simulink model "drone_1"  (R2024a)
settings: Solver=VariableStepAuto  StartTime=0.0  StopTime=10  RelTol=1e-3
model workspace: external: MATLAB File E:\MIT notes\SEM 5\DL PROJECT\ED_Lab_Project\drone_DataFile1.m (data not in the file)
undefined symbols (not defined in the file or in its folder): smiData, X, Y, Z
libraries: sm_lib x30, nesl_utility x13, fl_lib x10, simulink x1
settings Model: Creator=CAPTMKPC  LastModifiedBy=CAPTMKPC
settings ExplorerConfigSet: InternalSimMechanicsExplorerSettings="<ExplorerConfiguration><canonicalview>aerospace</canonicalview><AnimationSetting><BasePlaybackSpeed>1.0</BasePlaybackSpeed><PlaybackSpeedFactor>1.0</PlaybackSpeedFactor></AnimationSetting><TilePanel><TileInfo><Tiles Columns=\"1\" Count=\"1\" Rows=\"1\"><Column Weight=\"1\"/><Row Weight=\"1\"/><Tile Height=\"1\" Width=\"1\" X=\"0\" Y=\"0\"/></Tiles></TileInfo><SceneInfo><SceneViewer><BGColor><R>0.60000002384185791</R><G>0.60000002384185791</G><B>0.60000002384185791</B></BGColor><Camera><DoPerspective>off</DoPerspective><Position><X>1.8589269016645551</X><Y>0.22741887211799594</Y><Z>-0.0186989009380337107</Z></Position><Center><X>0.00202931501269310033</X><Y>0.22741887211799594</Y><Z>-0.0186989009380337107</Z></Center><Up><X>0</X><Y>0</Y><Z>-1</Z></Up><ViewLimDist>1</ViewLimDist><YLim>0.859905762768950144</YLim><XLim>1.52803398132324242</XLim></Camera></SceneViewer></SceneInfo></TilePanel><MechEditorPanel><Cameras/><GfxPanelCameraMap/><VideoCreator><PlaybackSpeedRatio>1.0</PlaybackSpeedRatio><FrameRate>30</FrameRate><VideoFormat>Motion JPEG AVI</VideoFormat><FrameSize>auto</FrameSize></VideoCreator></MechEditorPanel></ExplorerConfiguration>"

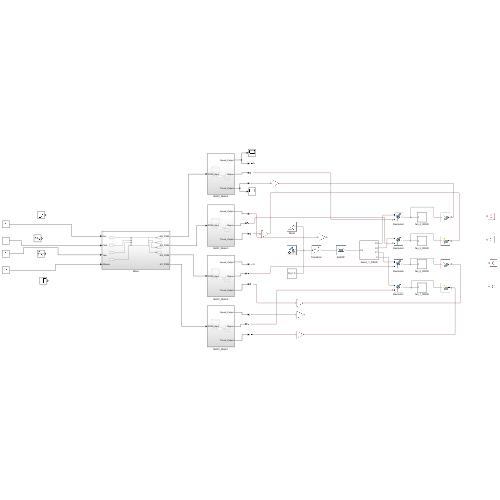
[thumbnail: Simulink's stored preview of the top-level diagram]
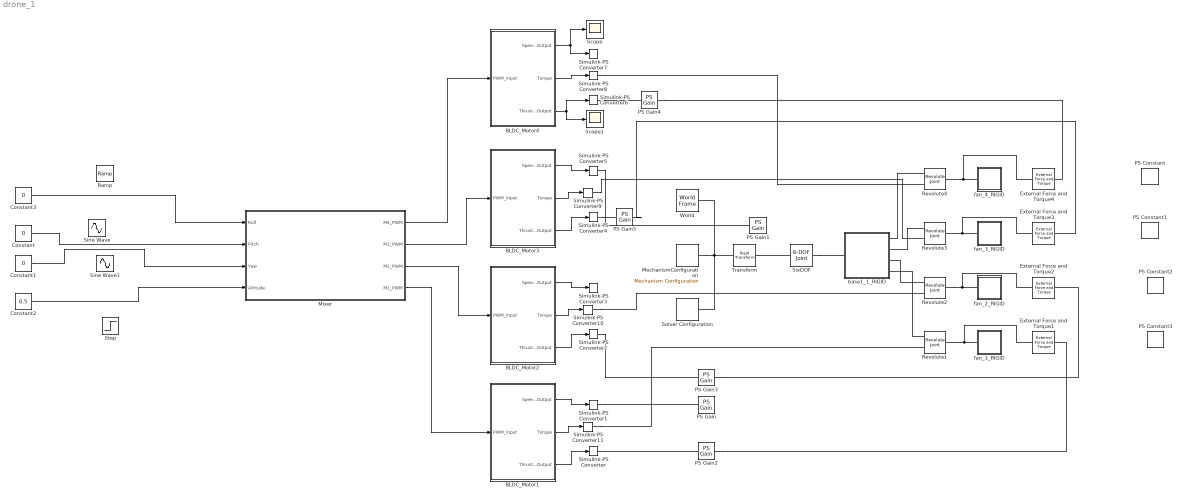
== system drone_1 ==
  BLDC_Motor1 : Subsystem
  BLDC_Motor2 : Subsystem
  BLDC_Motor3 : Subsystem
  BLDC_Motor4 : Subsystem
  Constant : Constant  Value=0
  Constant1 : Constant  Value=0
  Constant2 : Constant  Value=0.5
  Constant3 : Constant  Value=0
  External Force and Torque{1..4} (4 alike) : sm_lib/Forces and Torques/External Force and Torque  EnableForceX=off  EnableForceY=off  EnableForceZ=on  EnableForce=off  ForceResolutionFrame=World  EnableTorqueX=off  EnableTorqueY=off  EnableTorqueZ=off  EnableTorque=off  TorqueResolutionFrame=AttachedFrame
  MechanismConfiguration : sm_lib/Utilities/Mechanism Configuration  UniformGravity=Constant  GravityVector=[0 0 0]  GravityVectorUnits=m/s^2  LinearizationDelta=0.001  JointModeTransitionNonlinearIterations=2
  Mixer : Subsystem
  PS Constant{,1..3} (4 alike) : fl_lib/Physical Signals/Sources/PS Constant  constant=-308.4575 N
  PS Gain{,1..5} (6 alike) : fl_lib/Physical Signals/Functions/PS Gain  gain=-1
  Ramp : simulink/Sources/Ramp  slope=0.2  start=1  InitialOutput=0
  Revolute1 : sm_lib/Joints/Revolute Joint  JointMode=Normal  CompositeWrenchDir=FollowerOnBase  CompositeWrenchFrame=BaseFrame  SenseConstraintForce=off  SenseConstraintTorque=off  SenseTotalForce=off  SenseTotalTorque=off  PositionTargetSpecify=on  PositionTargetPriority=Low  PositionTargetValue=smiData.RevoluteJoint(1).Rz.Pos  PositionTargetValueUnits=deg  VelocityTargetSpecify=off  VelocityTargetPriority=High  VelocityTargetValue=0  VelocityTargetValueUnits=deg/s  EquilibriumPosition=0  EquilibriumPositionUnits=deg  SpringStiffness=0  SpringStiffnessUnits=N*m/deg  DampingCoefficient=0  DampingCoefficientUnits=N*m/(deg/s)  LowerLimitSpecify=off  LowerLimitBound=-90  LowerLimitBoundUnits=deg  LowerLimitStiffness=1e4  LowerLimitStiffnessUnits=N*m/deg  LowerLimitDamping=10  LowerLimitDampingUnits=N*m/(deg/s)  LowerLimitTransitionRegionWidth=0.1  LowerLimitTransitionRegionWidthUnits=deg  UpperLimitSpecify=off  UpperLimitBound=90  UpperLimitBoundUnits=deg  UpperLimitStiffness=1e4  UpperLimitStiffnessUnits=N*m/deg  UpperLimitDamping=10  UpperLimitDampingUnits=N*m/(deg/s)  UpperLimitTransitionRegionWidth=0.1  UpperLimitTransitionRegionWidthUnits=deg  TorqueActuationMode=InputTorque  MotionActuationMode=ComputedMotion  SensePosition=off  SenseVelocity=off  SenseAcceleration=off  SenseTorqueForce=off  SenseLowerLimitTorqueForce=off  SenseUpperLimitTorqueForce=off
  Revolute2 : sm_lib/Joints/Revolute Joint  JointMode=Normal  CompositeWrenchDir=FollowerOnBase  CompositeWrenchFrame=BaseFrame  SenseConstraintForce=off  SenseConstraintTorque=off  SenseTotalForce=off  SenseTotalTorque=off  PositionTargetSpecify=on  PositionTargetPriority=Low  PositionTargetValue=smiData.RevoluteJoint(2).Rz.Pos  PositionTargetValueUnits=deg  VelocityTargetSpecify=off  VelocityTargetPriority=High  VelocityTargetValue=0  VelocityTargetValueUnits=deg/s  EquilibriumPosition=0  EquilibriumPositionUnits=deg  SpringStiffness=0  SpringStiffnessUnits=N*m/deg  DampingCoefficient=0  DampingCoefficientUnits=N*m/(deg/s)  LowerLimitSpecify=off  LowerLimitBound=-90  LowerLimitBoundUnits=deg  LowerLimitStiffness=1e4  LowerLimitStiffnessUnits=N*m/deg  LowerLimitDamping=10  LowerLimitDampingUnits=N*m/(deg/s)  LowerLimitTransitionRegionWidth=0.1  LowerLimitTransitionRegionWidthUnits=deg  UpperLimitSpecify=off  UpperLimitBound=90  UpperLimitBoundUnits=deg  UpperLimitStiffness=1e4  UpperLimitStiffnessUnits=N*m/deg  UpperLimitDamping=10  UpperLimitDampingUnits=N*m/(deg/s)  UpperLimitTransitionRegionWidth=0.1  UpperLimitTransitionRegionWidthUnits=deg  TorqueActuationMode=InputTorque  MotionActuationMode=ComputedMotion  SensePosition=off  SenseVelocity=off  SenseAcceleration=off  SenseTorqueForce=off  SenseLowerLimitTorqueForce=off  SenseUpperLimitTorqueForce=off
  Revolute3 : sm_lib/Joints/Revolute Joint  JointMode=Normal  CompositeWrenchDir=FollowerOnBase  CompositeWrenchFrame=BaseFrame  SenseConstraintForce=off  SenseConstraintTorque=off  SenseTotalForce=off  SenseTotalTorque=off  PositionTargetSpecify=on  PositionTargetPriority=Low  PositionTargetValue=smiData.RevoluteJoint(3).Rz.Pos  PositionTargetValueUnits=deg  VelocityTargetSpecify=off  VelocityTargetPriority=High  VelocityTargetValue=0  VelocityTargetValueUnits=deg/s  EquilibriumPosition=0  EquilibriumPositionUnits=deg  SpringStiffness=0  SpringStiffnessUnits=N*m/deg  DampingCoefficient=0  DampingCoefficientUnits=N*m/(deg/s)  LowerLimitSpecify=off  LowerLimitBound=-90  LowerLimitBoundUnits=deg  LowerLimitStiffness=1e4  LowerLimitStiffnessUnits=N*m/deg  LowerLimitDamping=10  LowerLimitDampingUnits=N*m/(deg/s)  LowerLimitTransitionRegionWidth=0.1  LowerLimitTransitionRegionWidthUnits=deg  UpperLimitSpecify=off  UpperLimitBound=90  UpperLimitBoundUnits=deg  UpperLimitStiffness=1e4  UpperLimitStiffnessUnits=N*m/deg  UpperLimitDamping=10  UpperLimitDampingUnits=N*m/(deg/s)  UpperLimitTransitionRegionWidth=0.1  UpperLimitTransitionRegionWidthUnits=deg  TorqueActuationMode=InputTorque  MotionActuationMode=ComputedMotion  SensePosition=off  SenseVelocity=off  SenseAcceleration=off  SenseTorqueForce=off  SenseLowerLimitTorqueForce=off  SenseUpperLimitTorqueForce=off
  Revolute4 : sm_lib/Joints/Revolute Joint  JointMode=Normal  CompositeWrenchDir=FollowerOnBase  CompositeWrenchFrame=BaseFrame  SenseConstraintForce=off  SenseConstraintTorque=off  SenseTotalForce=off  SenseTotalTorque=off  PositionTargetSpecify=on  PositionTargetPriority=Low  PositionTargetValue=smiData.RevoluteJoint(4).Rz.Pos  PositionTargetValueUnits=deg  VelocityTargetSpecify=off  VelocityTargetPriority=High  VelocityTargetValue=0  VelocityTargetValueUnits=deg/s  EquilibriumPosition=0  EquilibriumPositionUnits=deg  SpringStiffness=0  SpringStiffnessUnits=N*m/deg  DampingCoefficient=0  DampingCoefficientUnits=N*m/(deg/s)  LowerLimitSpecify=off  LowerLimitBound=-90  LowerLimitBoundUnits=deg  LowerLimitStiffness=1e4  LowerLimitStiffnessUnits=N*m/deg  LowerLimitDamping=10  LowerLimitDampingUnits=N*m/(deg/s)  LowerLimitTransitionRegionWidth=0.1  LowerLimitTransitionRegionWidthUnits=deg  UpperLimitSpecify=off  UpperLimitBound=90  UpperLimitBoundUnits=deg  UpperLimitStiffness=1e4  UpperLimitStiffnessUnits=N*m/deg  UpperLimitDamping=10  UpperLimitDampingUnits=N*m/(deg/s)  UpperLimitTransitionRegionWidth=0.1  UpperLimitTransitionRegionWidthUnits=deg  TorqueActuationMode=InputTorque  MotionActuationMode=ComputedMotion  SensePosition=off  SenseVelocity=off  SenseAcceleration=off  SenseTorqueForce=off  SenseLowerLimitTorqueForce=off  SenseUpperLimitTorqueForce=off
  Scope : Scope
  Scope1 : Scope
  Simulink-PS Converter{,1..11} (12 alike) : nesl_utility/Simulink-PS Converter  PhysicalDomain=network_engine_domain  SubClassName=ps_input  LeftPortType=input  RightPortType=output  PseudoPeriodic=off  Frequencies=[]  NoiseDistribution=none  NoiseParameters=[]  Unit=1  AffineConversion=off  FilteringAndDerivatives=zero  SimscapeFilterOrder=1  InputFilterTimeConstant=0.001  UdotUserProvided=0
  Sine Wave : Sin  Amplitude=0.3  SampleTime=0
  Sine Wave1 : Sin  Amplitude=0.3  Frequency=0.5  Phase=90  SampleTime=0
  SixDOF : sm_lib/Joints/6-DOF Joint  JointMode=Normal  CompositeWrenchDir=FollowerOnBase  CompositeWrenchFrame=BaseFrame  SenseConstraintForce=off  SenseConstraintTorque=off  SenseTotalForce=off  SenseTotalTorque=off  PxPositionTargetSpecify=off  PxPositionTargetPriority=High  PxPositionTargetValue=0  PxPositionTargetValueUnits=m  PxVelocityTargetSpecify=off  PxVelocityTargetPriority=High  PxVelocityTargetValue=0  PxVelocityTargetValueUnits=m/s  PxEquilibriumPosition=0  PxEquilibriumPositionUnits=m  PxSpringStiffness=0  PxSpringStiffnessUnits=N/m  PxDampingCoefficient=0  PxDampingCoefficientUnits=N/(m/s)  PxLowerLimitSpecify=off  PxLowerLimitBound=-1  PxLowerLimitBoundUnits=m  PxLowerLimitStiffness=1e6  PxLowerLimitStiffnessUnits=N/m  PxLowerLimitDamping=1e3  PxLowerLimitDampingUnits=N/(m/s)  PxLowerLimitTransitionRegionWidth=1e-4  PxLowerLimitTransitionRegionWidthUnits=m  PxUpperLimitSpecify=off  PxUpperLimitBound=1  PxUpperLimitBoundUnits=m  PxUpperLimitStiffness=1e6  PxUpperLimitStiffnessUnits=N/m  PxUpperLimitDamping=1e3  PxUpperLimitDampingUnits=N/(m/s)  PxUpperLimitTransitionRegionWidth=1e-4  PxUpperLimitTransitionRegionWidthUnits=m  PxTorqueActuationMode=NoTorque  PxMotionActuationMode=ComputedMotion  PxSensePosition=off  PxSenseVelocity=off  PxSenseAcceleration=off  PxSenseTorqueForce=off  PxSenseLowerLimitTorqueForce=off  PxSenseUpperLimitTorqueForce=off  PyPositionTargetSpecify=off  PyPositionTargetPriority=High  PyPositionTargetValue=0  PyPositionTargetValueUnits=m  PyVelocityTargetSpecify=off  PyVelocityTargetPriority=High  PyVelocityTargetValue=0  PyVelocityTargetValueUnits=m/s  PyEquilibriumPosition=0  PyEquilibriumPositionUnits=m  PySpringStiffness=0  PySpringStiffnessUnits=N/m  PyDampingCoefficient=0  PyDampingCoefficientUnits=N/(m/s)  PyLowerLimitSpecify=off  PyLowerLimitBound=-1  PyLowerLimitBoundUnits=m  PyLowerLimitStiffness=1e6  PyLowerLimitStiffnessUnits=N/m  PyLowerLimitDamping=1e3  PyLowerLimitDampingUnits=N/(m/s)  PyLowerLimitTransitionRegionWidth=1e-4  PyLowerLimitTransitionRegionWidthUnits=m  PyUpperLimitSpecify=off  PyUpperLimitBound=1  PyUpperLimitBoundUnits=m  PyUpperLimitStiffness=1e6  PyUpperLimitStiffnessUnits=N/m  PyUpperLimitDamping=1e3  PyUpperLimitDampingUnits=N/(m/s)  PyUpperLimitTransitionRegionWidth=1e-4  PyUpperLimitTransitionRegionWidthUnits=m  PyTorqueActuationMode=NoTorque  PyMotionActuationMode=ComputedMotion  PySensePosition=off  PySenseVelocity=off  PySenseAcceleration=off  PySenseTorqueForce=off  PySenseLowerLimitTorqueForce=off  PySenseUpperLimitTorqueForce=off  PzPositionTargetSpecify=off  PzPositionTargetPriority=High  PzPositionTargetValue=0  PzPositionTargetValueUnits=m  PzVelocityTargetSpecify=off  PzVelocityTargetPriority=High  PzVelocityTargetValue=0  PzVelocityTargetValueUnits=m/s  PzEquilibriumPosition=0  PzEquilibriumPositionUnits=m  PzSpringStiffness=0  PzSpringStiffnessUnits=N/m  PzDampingCoefficient=0  PzDampingCoefficientUnits=N/(m/s)  PzLowerLimitSpecify=off  PzLowerLimitBound=-1  PzLowerLimitBoundUnits=m  PzLowerLimitStiffness=1e6  PzLowerLimitStiffnessUnits=N/m  PzLowerLimitDamping=1e3  PzLowerLimitDampingUnits=N/(m/s)  PzLowerLimitTransitionRegionWidth=1e-4  PzLowerLimitTransitionRegionWidthUnits=m  PzUpperLimitSpecify=off  PzUpperLimitBound=1  PzUpperLimitBoundUnits=m  PzUpperLimitStiffness=1e6  PzUpperLimitStiffnessUnits=N/m  PzUpperLimitDamping=1e3  PzUpperLimitDampingUnits=N/(m/s)  PzUpperLimitTransitionRegionWidth=1e-4  PzUpperLimitTransitionRegionWidthUnits=m  PzTorqueActuationMode=NoTorque  PzMotionActuationMode=ComputedMotion  PzSensePosition=off  PzSenseVelocity=off  PzSenseAcceleration=off  PzSenseTorqueForce=off  PzSenseLowerLimitTorqueForce=off  PzSenseUpperLimitTorqueForce=off  SphPositionTargetSpecify=off  SphPositionTargetPriority=High  SphPositionTargetRotationMethod=None  SphPositionTargetFollAlignAxisA=+X  SphPositionTargetBaseAlignAxisA=+Y  SphPositionTargetFollAlignAxisB=+Y  SphPositionTargetBaseAlignAxisB=+Z  SphPositionTargetRotationStandardAxis=+Z  SphPositionTargetRotationAngle=0  SphPositionTargetRotationAngleUnits=deg  SphPositionTargetRotationArbitraryAxis=[0 0 1]  SphPositionTargetRotationSequenceAxes=FollowerAxes  SphPositionTargetRotationSequence=XYX  SphPositionTargetRotationSequenceAngles=[0 0 0]  SphPositionTargetRotationSequenceAnglesUnits=deg  SphPositionTargetRotationMatrix=[1 0 0;0 1 0;0 0 1]  SphPositionTargetQuaternion=[1 0 0 0]  SphVelocityTargetSpecify=off  SphVelocityTargetPriority=High  SphVelocityTargetValue=[0 0 0]  SphVelocityTargetValueUnits=deg/s  SphVelocityTargetInFollowerFrame=on  SphEqPosRotationMethod=None  SphEqPosFollAlignAxisA=+X  SphEqPosBaseAlignAxisA=+Y  SphEqPosFollAlignAxisB=+Y  SphEqPosBaseAlignAxisB=+Z  SphEqPosRotationStandardAxis=+Z  SphEqPosRotationAngle=0  SphEqPosRotationAngleUnits=deg  SphEqPosRotationArbitraryAxis=[0 0 1]  SphEqPosRotationSequenceAxes=FollowerAxes  SphEqPosRotationSequence=XYX  SphEqPosRotationSequenceAngles=[0 0 0]  SphEqPosRotationSequenceAnglesUnits=deg  SphEqPosRotationMatrix=[1 0 0;0 1 0;0 0 1]  SphEqPosQuaternion=[1 0 0 0]  SphSpringStiffness=0  SphSpringStiffnessUnits=N*m/deg  SphDampingCoefficient=0  SphDampingCoefficientUnits=N*m/(deg/s)  SphLowerLimitSpecify=off  SphLowerLimitBound=15  SphLowerLimitBoundUnits=deg  SphLowerLimitStiffness=1e4  SphLowerLimitStiffnessUnits=N*m/deg  SphLowerLimitDamping=10  SphLowerLimitDampingUnits=N*m/(deg/s)  SphLowerLimitTransitionRegionWidth=0.1  SphLowerLimitTransitionRegionWidthUnits=deg  SphUpperLimitSpecify=off  SphUpperLimitBound=45  SphUpperLimitBoundUnits=deg  SphUpperLimitStiffness=1e4  SphUpperLimitStiffnessUnits=N*m/deg  SphUpperLimitDamping=10  SphUpperLimitDampingUnits=N*m/(deg/s)  SphUpperLimitTransitionRegionWidth=0.1  SphUpperLimitTransitionRegionWidthUnits=deg  SphTorqueActuationMode=NoTorque  SphActuateTorqueX=off  SphActuateTorqueY=off  SphActuateTorqueZ=off  SphActuateTorque=off  SphActuationFrame=BaseFrame  SphSensePosition=off  SphSenseVelocityX=off  SphSenseVelocityY=off  SphSenseVelocityZ=off  SphSenseVelocity=off  SphSenseAccelerationX=off  SphSenseAccelerationY=off  SphSenseAccelerationZ=off  SphSenseAcceleration=off  SphSenseLowerLimitTorqueMag=off  SphSenseUpperLimitTorqueMag=off  SphSensingFrame=FollowerFrame
  Solver Configuration : nesl_utility/Solver Configuration  PhysicalDomain=network_engine_domain  SubClassName=solver  LeftPortType=input  RightPortType=generic  Tones=[]  Harmonics=[]  SimulateNoise=off  Profile=off  UseLocalSampling=off  EnableSwitchedLinearOptims=on  FrequencyDomain=off  UseCCode=off  RelTol=0.001  AbsTol=0.001  MinStep=1e-09  ToWorkspace=off  RevertToSquareIcSolve=off  NumHomotopyIterations=100  PhasorMode=off  PhasorModeNumHarmonics=1  ConsistencySolver=NEWTON_XTOL_AFTER_FTOL  IndexReductionMethod=DerivativeReplacement  DoDC=off  ResidualTolerance=1e-09  ConsistencyTolSource=GLOBAL  ConsistencyAbsTol=0.001  ConsistencyRelTol=0.001  ConsistencyTolFactor=0.001  UseLocalSolver=off  LocalSolverChoice=NE_BACKWARD_EULER_ADVANCER  ResolveIndetEquations=on  FunctionEvalNumThread=1  LocalSolverSampleTime=0.001  DoFixedCost=off  MaxNonlinIter=3  MaxModeIter=2  ComputeImpulses=off  ImpulseIterations=2  LinearAlgebra=auto  LinearAlgebraNumThread=0  EquationFormulation=NE_TIME_EF  DelaysMemoryBudget=1024  AutomaticFiltering=on  FilteringTimeConstant=0.001  PartitionStorageMethod=AS_NEEDED  PartitionMemoryBudget=1024  PartitionMethod=ROBUST  MultibodyUseLocalSolver=off  MultibodyLocalSolverChoice=ODE1  MultibodyLocalSolverSampleTime=0.001
  Step : Step  Time=3  After=0.2  SampleTime=0
  Transform : sm_lib/Frames and Transforms/Rigid Transform  RotationMethod=StandardAxis  FollAlignAxisA=+X  BaseAlignAxisA=+Y  FollAlignAxisB=+Y  BaseAlignAxisB=+Z  RotationStandardAxis=+X  RotationAngle=-90  RotationAngleUnits=deg  RotationArbitraryAxis=smiData.RigidTransform(9).axis  RotationSequenceAxes=FollowerAxes  RotationSequence=XYX  RotationSequenceAngles=[0 0 0]  RotationSequenceAnglesUnits=deg  RotationMatrix=[1 0 0;0 1 0;0 0 1]  Quaternion=[1 0 0 0]  TranslationMethod=Cartesian  TranslationCartesianOffset=smiData.RigidTransform(9).translation  TranslationCartesianOffsetUnits=mm  TranslationStandardAxis=+Z  TranslationStandardOffset=0  TranslationStandardOffsetUnits=m  TranslationROffset=0  TranslationROffsetUnits=m  TranslationThetaOffset=0  TranslationThetaOffsetUnits=deg  TranslationZOffset=0  TranslationZOffsetUnits=m
  World : sm_lib/Frames and Transforms/World Frame
  base1_1_RIGID : Subsystem
  fan_1_RIGID : Subsystem
  fan_2_RIGID : Subsystem
  fan_3_RIGID : Subsystem
  fan_4_RIGID : Subsystem
  wires:
  BLDC_Motor4/1(Speed_Output) -> Simulink-PS Converter7/1, Scope/1
  BLDC_Motor4/3(Thrust_Output) -> Simulink-PS Converter6/1, Scope1/1
  Mixer/1(M4_PWM) -> BLDC_Motor4/1(PWM_Input)
  Constant3/1 -> Mixer/1(Roll)
  Constant/1 -> Mixer/2(Pitch)
  Constant1/1 -> Mixer/3(Yaw)
  Constant2/1 -> Mixer/4(Altitude)
  BLDC_Motor3/1(Speed_Output) -> Simulink-PS Converter5/1
  BLDC_Motor3/3(Thrust_Output) -> Simulink-PS Converter4/1
  BLDC_Motor2/1(Speed_Output) -> Simulink-PS Converter3/1
  BLDC_Motor2/3(Thrust_Output) -> Simulink-PS Converter2/1
  BLDC_Motor1/1(Speed_Output) -> Simulink-PS Converter1/1
  BLDC_Motor1/3(Thrust_Output) -> Simulink-PS Converter/1
  Mixer/2(M3_PWM) -> BLDC_Motor3/1(PWM_Input)
  Mixer/3(M2_PWM) -> BLDC_Motor2/1(PWM_Input)
  Mixer/4(M1_PWM) -> BLDC_Motor1/1(PWM_Input)
  BLDC_Motor4/2(Torque) -> Simulink-PS Converter8/1
  BLDC_Motor3/2(Torque) -> Simulink-PS Converter9/1
  BLDC_Motor2/2(Torque) -> Simulink-PS Converter10/1
  BLDC_Motor1/2(Torque) -> Simulink-PS Converter11/1
  connections:
  MechanismConfiguration/RConn1 -- Solver Configuration/RConn1 -- Transform/LConn1 -- World/RConn1
  Revolute1/LConn1 -- base1_1_RIGID/RConn4
  SixDOF/LConn1 -- Transform/RConn1
  Revolute1/RConn1 -- External Force and Torque1/RConn1 -- fan_1_RIGID/LConn1
  Revolute2/LConn1 -- base1_1_RIGID/RConn3
  Revolute2/RConn1 -- External Force and Torque2/RConn1 -- fan_2_RIGID/LConn1
  Revolute3/LConn1 -- base1_1_RIGID/RConn2
  Revolute3/RConn1 -- External Force and Torque3/RConn1 -- fan_3_RIGID/LConn1
  Revolute4/LConn1 -- base1_1_RIGID/RConn1
  Revolute4/RConn1 -- External Force and Torque4/RConn1 -- fan_4_RIGID/LConn1
  SixDOF/RConn1 -- base1_1_RIGID/LConn1
  Simulink-PS Converter6/RConn1 -- PS Gain4/LConn1
  Simulink-PS Converter4/RConn1 -- PS Gain5/LConn1
  Simulink-PS Converter2/RConn1 -- PS Gain3/LConn1
  Simulink-PS Converter/RConn1 -- PS Gain2/LConn1
  Simulink-PS Converter5/RConn1 -- PS Gain1/LConn1
  Simulink-PS Converter1/RConn1 -- PS Gain/LConn1
  PS Gain2/RConn1 -- External Force and Torque1/LConn1
  PS Gain3/RConn1 -- External Force and Torque2/LConn1
  PS Gain4/RConn1 -- External Force and Torque4/LConn1
  PS Gain5/RConn1 -- External Force and Torque3/LConn1
  Simulink-PS Converter8/RConn1 -- Revolute4/LConn2
  Simulink-PS Converter9/RConn1 -- Revolute3/LConn2
  Simulink-PS Converter10/RConn1 -- Revolute2/LConn2
  Simulink-PS Converter11/RConn1 -- Revolute1/LConn2

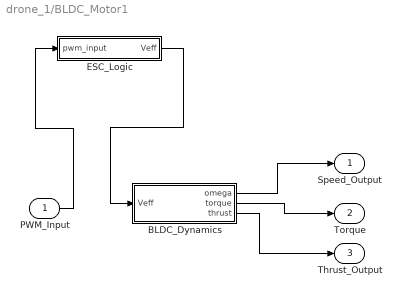
== system drone_1/BLDC_Motor1 ==
  PWM_Input : Inport
  BLDC_Dynamics : MATLAB Function  TreatAsAtomicUnit=on
  ESC_Logic : MATLAB Function  TreatAsAtomicUnit=on
  Speed_Output : Outport
  Torque : Outport  Port=2
  Thrust_Output : Outport  Port=3
  wires:
  BLDC_Dynamics/2(torque) -> Torque/1
  BLDC_Dynamics/1(omega) -> Speed_Output/1
  BLDC_Dynamics/3(thrust) -> Thrust_Output/1
  ESC_Logic/1(Veff) -> BLDC_Dynamics/1(Veff)
  PWM_Input/1 -> ESC_Logic/1(pwm_input)

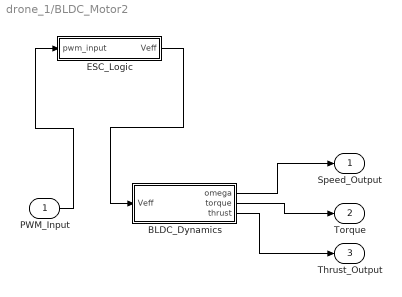
== system drone_1/BLDC_Motor2 ==
  PWM_Input : Inport
  BLDC_Dynamics : MATLAB Function  TreatAsAtomicUnit=on
  ESC_Logic : MATLAB Function  TreatAsAtomicUnit=on
  Speed_Output : Outport
  Torque : Outport  Port=2
  Thrust_Output : Outport  Port=3
  wires:
  BLDC_Dynamics/2(torque) -> Torque/1
  BLDC_Dynamics/1(omega) -> Speed_Output/1
  BLDC_Dynamics/3(thrust) -> Thrust_Output/1
  ESC_Logic/1(Veff) -> BLDC_Dynamics/1(Veff)
  PWM_Input/1 -> ESC_Logic/1(pwm_input)

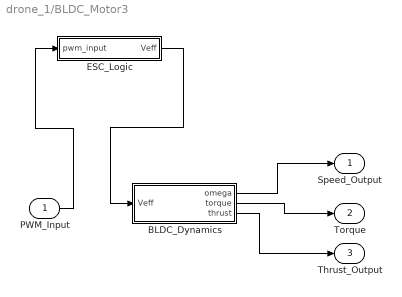
== system drone_1/BLDC_Motor3 ==
  PWM_Input : Inport
  BLDC_Dynamics : MATLAB Function  TreatAsAtomicUnit=on
  ESC_Logic : MATLAB Function  TreatAsAtomicUnit=on
  Speed_Output : Outport
  Torque : Outport  Port=2
  Thrust_Output : Outport  Port=3
  wires:
  BLDC_Dynamics/2(torque) -> Torque/1
  BLDC_Dynamics/1(omega) -> Speed_Output/1
  BLDC_Dynamics/3(thrust) -> Thrust_Output/1
  ESC_Logic/1(Veff) -> BLDC_Dynamics/1(Veff)
  PWM_Input/1 -> ESC_Logic/1(pwm_input)

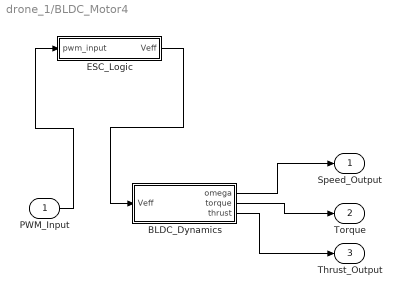
== system drone_1/BLDC_Motor4 ==
  PWM_Input : Inport
  BLDC_Dynamics : MATLAB Function  TreatAsAtomicUnit=on
  ESC_Logic : MATLAB Function  TreatAsAtomicUnit=on
  Speed_Output : Outport
  Torque : Outport  Port=2
  Thrust_Output : Outport  Port=3
  wires:
  ESC_Logic/1(Veff) -> BLDC_Dynamics/1(Veff)
  PWM_Input/1 -> ESC_Logic/1(pwm_input)
  BLDC_Dynamics/1(omega) -> Speed_Output/1
  BLDC_Dynamics/2(torque) -> Torque/1
  BLDC_Dynamics/3(thrust) -> Thrust_Output/1

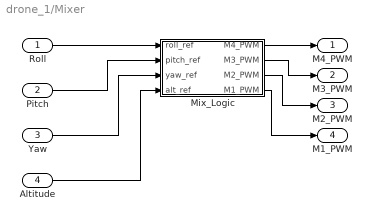
== system drone_1/Mixer ==
  Roll : Inport
  Pitch : Inport  Port=2
  Yaw : Inport  Port=3
  Altitude : Inport  Port=4
  Mix_Logic : MATLAB Function  TreatAsAtomicUnit=on
  M4_PWM : Outport
  M3_PWM : Outport  Port=2
  M2_PWM : Outport  Port=3
  M1_PWM : Outport  Port=4
  wires:
  Roll/1 -> Mix_Logic/1(roll_ref)
  Pitch/1 -> Mix_Logic/2(pitch_ref)
  Yaw/1 -> Mix_Logic/3(yaw_ref)
  Mix_Logic/1(M4_PWM) -> M4_PWM/1
  Mix_Logic/2(M3_PWM) -> M3_PWM/1
  Mix_Logic/3(M2_PWM) -> M2_PWM/1
  Mix_Logic/4(M1_PWM) -> M1_PWM/1
  Altitude/1 -> Mix_Logic/4(alt_ref)

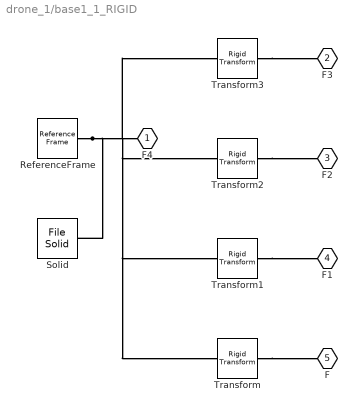
== system drone_1/base1_1_RIGID ==
  ReferenceFrame : sm_lib/Frames and Transforms/Reference Frame
  Solid : sm_lib/Body Elements/File Solid  ExtGeomFileName=base1_Default_sldprt.STEP  UnitType=FromFile  ExtGeomFileUnits=m  StepReaderType=HEX  ExportConvexHullGeometry=off  InertiaType=Custom  BasedOnType=DensityFromFile  Density=1000  DensityUnits=kg/m^3  Mass=smiData.Solid(1).mass  MassUnits=kg  CenterOfMass=smiData.Solid(1).CoM  CenterOfMassUnits=mm  MomentsOfInertia=smiData.Solid(1).MoI  MomentsOfInertiaUnits=kg*mm^2  ProductsOfInertia=smiData.Solid(1).PoI  ProductsOfInertiaUnits=kg*mm^2  GraphicType=FromGeometry  MarkerShape=Sphere  MarkerSize=10  GraphicVisPropType=SimpleVisualProperties  GraphicDiffuseColor=smiData.Solid(1).color  GraphicOpacity=smiData.Solid(1).opacity  GraphicSpecularColor=[0.5 0.5 0.5 1.0]  GraphicAmbientColor=[0.15 0.15 0.15 1.0]  GraphicEmissiveColor=[0.0 0.0 0.0 1.0]  GraphicShininess=75  DoExposeReferenceFrame=on  SerializedFrames=<Frames/>
  Transform : sm_lib/Frames and Transforms/Rigid Transform  RotationMethod=ArbitraryAxis  FollAlignAxisA=+X  BaseAlignAxisA=+Y  FollAlignAxisB=+Y  BaseAlignAxisB=+Z  RotationStandardAxis=+Z  RotationAngle=smiData.RigidTransform(1).angle  RotationAngleUnits=rad  RotationArbitraryAxis=smiData.RigidTransform(1).axis  RotationSequenceAxes=FollowerAxes  RotationSequence=XYX  RotationSequenceAngles=[0 0 0]  RotationSequenceAnglesUnits=deg  RotationMatrix=[1 0 0;0 1 0;0 0 1]  Quaternion=[1 0 0 0]  TranslationMethod=Cartesian  TranslationCartesianOffset=smiData.RigidTransform(1).translation  TranslationCartesianOffsetUnits=mm  TranslationStandardAxis=+Z  TranslationStandardOffset=0  TranslationStandardOffsetUnits=m  TranslationROffset=0  TranslationROffsetUnits=m  TranslationThetaOffset=0  TranslationThetaOffsetUnits=deg  TranslationZOffset=0  TranslationZOffsetUnits=m
  Transform1 : sm_lib/Frames and Transforms/Rigid Transform  RotationMethod=ArbitraryAxis  FollAlignAxisA=+X  BaseAlignAxisA=+Y  FollAlignAxisB=+Y  BaseAlignAxisB=+Z  RotationStandardAxis=+Z  RotationAngle=smiData.RigidTransform(3).angle  RotationAngleUnits=rad  RotationArbitraryAxis=smiData.RigidTransform(3).axis  RotationSequenceAxes=FollowerAxes  RotationSequence=XYX  RotationSequenceAngles=[0 0 0]  RotationSequenceAnglesUnits=deg  RotationMatrix=[1 0 0;0 1 0;0 0 1]  Quaternion=[1 0 0 0]  TranslationMethod=Cartesian  TranslationCartesianOffset=smiData.RigidTransform(3).translation  TranslationCartesianOffsetUnits=mm  TranslationStandardAxis=+Z  TranslationStandardOffset=0  TranslationStandardOffsetUnits=m  TranslationROffset=0  TranslationROffsetUnits=m  TranslationThetaOffset=0  TranslationThetaOffsetUnits=deg  TranslationZOffset=0  TranslationZOffsetUnits=m
  Transform2 : sm_lib/Frames and Transforms/Rigid Transform  RotationMethod=ArbitraryAxis  FollAlignAxisA=+X  BaseAlignAxisA=+Y  FollAlignAxisB=+Y  BaseAlignAxisB=+Z  RotationStandardAxis=+Z  RotationAngle=smiData.RigidTransform(5).angle  RotationAngleUnits=rad  RotationArbitraryAxis=smiData.RigidTransform(5).axis  RotationSequenceAxes=FollowerAxes  RotationSequence=XYX  RotationSequenceAngles=[0 0 0]  RotationSequenceAnglesUnits=deg  RotationMatrix=[1 0 0;0 1 0;0 0 1]  Quaternion=[1 0 0 0]  TranslationMethod=Cartesian  TranslationCartesianOffset=smiData.RigidTransform(5).translation  TranslationCartesianOffsetUnits=mm  TranslationStandardAxis=+Z  TranslationStandardOffset=0  TranslationStandardOffsetUnits=m  TranslationROffset=0  TranslationROffsetUnits=m  TranslationThetaOffset=0  TranslationThetaOffsetUnits=deg  TranslationZOffset=0  TranslationZOffsetUnits=m
  Transform3 : sm_lib/Frames and Transforms/Rigid Transform  RotationMethod=ArbitraryAxis  FollAlignAxisA=+X  BaseAlignAxisA=+Y  FollAlignAxisB=+Y  BaseAlignAxisB=+Z  RotationStandardAxis=+Z  RotationAngle=smiData.RigidTransform(7).angle  RotationAngleUnits=rad  RotationArbitraryAxis=smiData.RigidTransform(7).axis  RotationSequenceAxes=FollowerAxes  RotationSequence=XYX  RotationSequenceAngles=[0 0 0]  RotationSequenceAnglesUnits=deg  RotationMatrix=[1 0 0;0 1 0;0 0 1]  Quaternion=[1 0 0 0]  TranslationMethod=Cartesian  TranslationCartesianOffset=smiData.RigidTransform(7).translation  TranslationCartesianOffsetUnits=mm  TranslationStandardAxis=+Z  TranslationStandardOffset=0  TranslationStandardOffsetUnits=m  TranslationROffset=0  TranslationROffsetUnits=m  TranslationThetaOffset=0  TranslationThetaOffsetUnits=deg  TranslationZOffset=0  TranslationZOffsetUnits=m
  F4 : PMIOPort  Side=Left
  F3 : PMIOPort  Port=2  Side=Right
  F2 : PMIOPort  Port=3  Side=Right
  F1 : PMIOPort  Port=4  Side=Right
  F : PMIOPort  Port=5  Side=Right
  connections:
  Solid/RConn1 -- ReferenceFrame/RConn1 -- Transform/LConn1 -- Transform1/LConn1 -- Transform2/LConn1 -- Transform3/LConn1 -- F4/RConn1
  Transform/RConn1 -- F/RConn1
  Transform1/RConn1 -- F1/RConn1
  Transform2/RConn1 -- F2/RConn1
  Transform3/RConn1 -- F3/RConn1

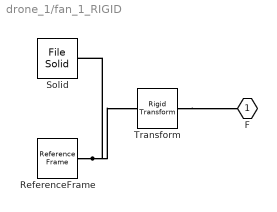
== system drone_1/fan_1_RIGID ==
  ReferenceFrame : sm_lib/Frames and Transforms/Reference Frame
  Solid : sm_lib/Body Elements/File Solid  ExtGeomFileName=fan_Default_sldprt.STEP  UnitType=FromFile  ExtGeomFileUnits=m  StepReaderType=HEX  ExportConvexHullGeometry=off  InertiaType=Custom  BasedOnType=DensityFromFile  Density=1000  DensityUnits=kg/m^3  Mass=smiData.Solid(2).mass  MassUnits=kg  CenterOfMass=smiData.Solid(2).CoM  CenterOfMassUnits=mm  MomentsOfInertia=smiData.Solid(2).MoI  MomentsOfInertiaUnits=kg*mm^2  ProductsOfInertia=smiData.Solid(2).PoI  ProductsOfInertiaUnits=kg*mm^2  GraphicType=FromGeometry  MarkerShape=Sphere  MarkerSize=10  GraphicVisPropType=SimpleVisualProperties  GraphicDiffuseColor=smiData.Solid(2).color  GraphicOpacity=smiData.Solid(2).opacity  GraphicSpecularColor=[0.5 0.5 0.5 1.0]  GraphicAmbientColor=[0.15 0.15 0.15 1.0]  GraphicEmissiveColor=[0.0 0.0 0.0 1.0]  GraphicShininess=75  DoExposeReferenceFrame=on  SerializedFrames=<Frames/>
  Transform : sm_lib/Frames and Transforms/Rigid Transform  RotationMethod=ArbitraryAxis  FollAlignAxisA=+X  BaseAlignAxisA=+Y  FollAlignAxisB=+Y  BaseAlignAxisB=+Z  RotationStandardAxis=+Z  RotationAngle=smiData.RigidTransform(2).angle  RotationAngleUnits=rad  RotationArbitraryAxis=smiData.RigidTransform(2).axis  RotationSequenceAxes=FollowerAxes  RotationSequence=XYX  RotationSequenceAngles=[0 0 0]  RotationSequenceAnglesUnits=deg  RotationMatrix=[1 0 0;0 1 0;0 0 1]  Quaternion=[1 0 0 0]  TranslationMethod=Cartesian  TranslationCartesianOffset=smiData.RigidTransform(2).translation  TranslationCartesianOffsetUnits=mm  TranslationStandardAxis=+Z  TranslationStandardOffset=0  TranslationStandardOffsetUnits=m  TranslationROffset=0  TranslationROffsetUnits=m  TranslationThetaOffset=0  TranslationThetaOffsetUnits=deg  TranslationZOffset=0  TranslationZOffsetUnits=m
  F : PMIOPort  Side=Left
  connections:
  Solid/RConn1 -- ReferenceFrame/RConn1 -- Transform/LConn1
  Transform/RConn1 -- F/RConn1

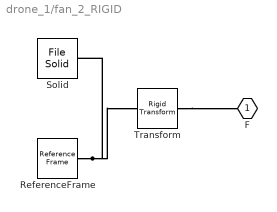
== system drone_1/fan_2_RIGID ==
  ReferenceFrame : sm_lib/Frames and Transforms/Reference Frame
  Solid : sm_lib/Body Elements/File Solid  ExtGeomFileName=fan_Default_sldprt.STEP  UnitType=FromFile  ExtGeomFileUnits=m  StepReaderType=HEX  ExportConvexHullGeometry=off  InertiaType=Custom  BasedOnType=DensityFromFile  Density=1000  DensityUnits=kg/m^3  Mass=smiData.Solid(2).mass  MassUnits=kg  CenterOfMass=smiData.Solid(2).CoM  CenterOfMassUnits=mm  MomentsOfInertia=smiData.Solid(2).MoI  MomentsOfInertiaUnits=kg*mm^2  ProductsOfInertia=smiData.Solid(2).PoI  ProductsOfInertiaUnits=kg*mm^2  GraphicType=FromGeometry  MarkerShape=Sphere  MarkerSize=10  GraphicVisPropType=SimpleVisualProperties  GraphicDiffuseColor=smiData.Solid(2).color  GraphicOpacity=smiData.Solid(2).opacity  GraphicSpecularColor=[0.5 0.5 0.5 1.0]  GraphicAmbientColor=[0.15 0.15 0.15 1.0]  GraphicEmissiveColor=[0.0 0.0 0.0 1.0]  GraphicShininess=75  DoExposeReferenceFrame=on  SerializedFrames=<Frames/>
  Transform : sm_lib/Frames and Transforms/Rigid Transform  RotationMethod=ArbitraryAxis  FollAlignAxisA=+X  BaseAlignAxisA=+Y  FollAlignAxisB=+Y  BaseAlignAxisB=+Z  RotationStandardAxis=+Z  RotationAngle=smiData.RigidTransform(4).angle  RotationAngleUnits=rad  RotationArbitraryAxis=smiData.RigidTransform(4).axis  RotationSequenceAxes=FollowerAxes  RotationSequence=XYX  RotationSequenceAngles=[0 0 0]  RotationSequenceAnglesUnits=deg  RotationMatrix=[1 0 0;0 1 0;0 0 1]  Quaternion=[1 0 0 0]  TranslationMethod=Cartesian  TranslationCartesianOffset=smiData.RigidTransform(4).translation  TranslationCartesianOffsetUnits=mm  TranslationStandardAxis=+Z  TranslationStandardOffset=0  TranslationStandardOffsetUnits=m  TranslationROffset=0  TranslationROffsetUnits=m  TranslationThetaOffset=0  TranslationThetaOffsetUnits=deg  TranslationZOffset=0  TranslationZOffsetUnits=m
  F : PMIOPort  Side=Left
  connections:
  Solid/RConn1 -- ReferenceFrame/RConn1 -- Transform/LConn1
  Transform/RConn1 -- F/RConn1

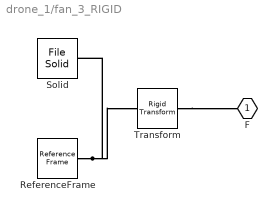
== system drone_1/fan_3_RIGID ==
  ReferenceFrame : sm_lib/Frames and Transforms/Reference Frame
  Solid : sm_lib/Body Elements/File Solid  ExtGeomFileName=fan_Default_sldprt.STEP  UnitType=FromFile  ExtGeomFileUnits=m  StepReaderType=HEX  ExportConvexHullGeometry=off  InertiaType=Custom  BasedOnType=DensityFromFile  Density=1000  DensityUnits=kg/m^3  Mass=smiData.Solid(2).mass  MassUnits=kg  CenterOfMass=smiData.Solid(2).CoM  CenterOfMassUnits=mm  MomentsOfInertia=smiData.Solid(2).MoI  MomentsOfInertiaUnits=kg*mm^2  ProductsOfInertia=smiData.Solid(2).PoI  ProductsOfInertiaUnits=kg*mm^2  GraphicType=FromGeometry  MarkerShape=Sphere  MarkerSize=10  GraphicVisPropType=SimpleVisualProperties  GraphicDiffuseColor=smiData.Solid(2).color  GraphicOpacity=smiData.Solid(2).opacity  GraphicSpecularColor=[0.5 0.5 0.5 1.0]  GraphicAmbientColor=[0.15 0.15 0.15 1.0]  GraphicEmissiveColor=[0.0 0.0 0.0 1.0]  GraphicShininess=75  DoExposeReferenceFrame=on  SerializedFrames=<Frames/>
  Transform : sm_lib/Frames and Transforms/Rigid Transform  RotationMethod=ArbitraryAxis  FollAlignAxisA=+X  BaseAlignAxisA=+Y  FollAlignAxisB=+Y  BaseAlignAxisB=+Z  RotationStandardAxis=+Z  RotationAngle=smiData.RigidTransform(6).angle  RotationAngleUnits=rad  RotationArbitraryAxis=smiData.RigidTransform(6).axis  RotationSequenceAxes=FollowerAxes  RotationSequence=XYX  RotationSequenceAngles=[0 0 0]  RotationSequenceAnglesUnits=deg  RotationMatrix=[1 0 0;0 1 0;0 0 1]  Quaternion=[1 0 0 0]  TranslationMethod=Cartesian  TranslationCartesianOffset=smiData.RigidTransform(6).translation  TranslationCartesianOffsetUnits=mm  TranslationStandardAxis=+Z  TranslationStandardOffset=0  TranslationStandardOffsetUnits=m  TranslationROffset=0  TranslationROffsetUnits=m  TranslationThetaOffset=0  TranslationThetaOffsetUnits=deg  TranslationZOffset=0  TranslationZOffsetUnits=m
  F : PMIOPort  Side=Left
  connections:
  Solid/RConn1 -- ReferenceFrame/RConn1 -- Transform/LConn1
  Transform/RConn1 -- F/RConn1

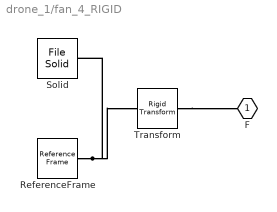
== system drone_1/fan_4_RIGID ==
  ReferenceFrame : sm_lib/Frames and Transforms/Reference Frame
  Solid : sm_lib/Body Elements/File Solid  ExtGeomFileName=fan_Default_sldprt.STEP  UnitType=FromFile  ExtGeomFileUnits=m  StepReaderType=HEX  ExportConvexHullGeometry=off  InertiaType=Custom  BasedOnType=DensityFromFile  Density=1000  DensityUnits=kg/m^3  Mass=smiData.Solid(2).mass  MassUnits=kg  CenterOfMass=smiData.Solid(2).CoM  CenterOfMassUnits=mm  MomentsOfInertia=smiData.Solid(2).MoI  MomentsOfInertiaUnits=kg*mm^2  ProductsOfInertia=smiData.Solid(2).PoI  ProductsOfInertiaUnits=kg*mm^2  GraphicType=FromGeometry  MarkerShape=Sphere  MarkerSize=10  GraphicVisPropType=SimpleVisualProperties  GraphicDiffuseColor=smiData.Solid(2).color  GraphicOpacity=smiData.Solid(2).opacity  GraphicSpecularColor=[0.5 0.5 0.5 1.0]  GraphicAmbientColor=[0.15 0.15 0.15 1.0]  GraphicEmissiveColor=[0.0 0.0 0.0 1.0]  GraphicShininess=75  DoExposeReferenceFrame=on  SerializedFrames=<Frames/>
  Transform : sm_lib/Frames and Transforms/Rigid Transform  RotationMethod=ArbitraryAxis  FollAlignAxisA=+X  BaseAlignAxisA=+Y  FollAlignAxisB=+Y  BaseAlignAxisB=+Z  RotationStandardAxis=+Z  RotationAngle=smiData.RigidTransform(8).angle  RotationAngleUnits=rad  RotationArbitraryAxis=smiData.RigidTransform(8).axis  RotationSequenceAxes=FollowerAxes  RotationSequence=XYX  RotationSequenceAngles=[0 0 0]  RotationSequenceAnglesUnits=deg  RotationMatrix=[1 0 0;0 1 0;0 0 1]  Quaternion=[1 0 0 0]  TranslationMethod=Cartesian  TranslationCartesianOffset=smiData.RigidTransform(8).translation  TranslationCartesianOffsetUnits=mm  TranslationStandardAxis=+Z  TranslationStandardOffset=0  TranslationStandardOffsetUnits=m  TranslationROffset=0  TranslationROffsetUnits=m  TranslationThetaOffset=0  TranslationThetaOffsetUnits=deg  TranslationZOffset=0  TranslationZOffsetUnits=m
  F : PMIOPort  Side=Left
  connections:
  Solid/RConn1 -- ReferenceFrame/RConn1 -- Transform/LConn1
  Transform/RConn1 -- F/RConn1

== matlab function drone_1/BLDC_Motor1/BLDC_Dynamics ==
  settings: updateMethod=DISCRETE
  data: Veff input; omega output; torque output; thrust output
function [omega, torque, thrust] = fcn(Veff)
%#codegen
% Simplified BLDC Motor and Propeller Dynamics for Quadcopter
% Input:
%   Veff - Effective voltage from ESC (V)
% Outputs:
%   omega - Motor angular velocity (rad/s)
%   torque - Motor torque (N*m)
%   thrust - Propeller thrust (N)

% Motor Parameters (based on your drone mass and inertia data)
Kv = 920;                  % Motor velocity constant (RPM/V)
Km = 60/(Kv*2*pi);        % Motor torque constant (N*m/A)
R = 0.1;                  % Motor resistance (ohm)
J = 1.915e-3;            % Rotor inertia from provided data (kg*m^2)
B = 1e-5;                % Viscous damping coefficient (N*m*s)

% Propeller Parameters
Ct = 1.2e-6;             % Thrust coefficient
Cq = 1.8e-7;             % Torque coefficient
rho = 1.225;             % Air density (kg/m^3)
D = 0.254;               % Propeller diameter (m)

% Motor Speed Calculation
% Using steady-state approximation
omega = (Veff - 0)/(Km^2/R + B);  % Steady state speed

% Torque Calculation
current = (Veff - Km*omega)/R;
aero_torque = Cq*rho*D^5*omega^2;
torque = Km*current - B*omega - aero_torque;

% Thrust Calculation
thrust = Ct*rho*D^4*omega^2;

% Limit minimum speed/thrust for numerical stability
if omega < 0
    omega = 0;
    torque = 0;
    thrust = 0;
end
end

== matlab function drone_1/BLDC_Motor1/ESC_Logic ==
  data: pwm_input input; Veff output
function Veff = fcn(pwm_input)
%#codegen
% Simplified ESC Logic for BLDC Motor Control
% Input:
%   pwm_input - PWM signal (0 to 1)
% Output:
%   Veff - Effective voltage to motor (V)

% ESC Parameters
MIN_THROTTLE = 0.05;        % Minimum throttle (deadband)
MAX_THROTTLE = 0.95;        % Maximum throttle limit
BATTERY_VOLTAGE = 14.8;     % Assuming 4S LiPo (14.8V)

% Apply deadband
if pwm_input < MIN_THROTTLE
    normalized_pwm = 0;
elseif pwm_input > MAX_THROTTLE
    normalized_pwm = 1;
else
    % Normalize PWM to 0-1 range considering deadband
    normalized_pwm = (pwm_input - MIN_THROTTLE) / (MAX_THROTTLE - MIN_THROTTLE);
end

% Convert to effective voltage
Veff = BATTERY_VOLTAGE * normalized_pwm;
end

== matlab function drone_1/Mixer/Mix_Logic ==
  data: M4_PWM output; M3_PWM output; M2_PWM output; roll_ref input; M1_PWM output; pitch_ref input; yaw_ref input; alt_ref input
function [M4_PWM, M3_PWM, M2_PWM, M1_PWM] = fcn(roll_ref, pitch_ref, yaw_ref, alt_ref)
%#codegen
% This function implements a motor mixer for a quadcopter with X configuration
% Inputs:
%   roll_ref  - Roll reference command (-1 to 1)
%   pitch_ref - Pitch reference command (-1 to 1)
%   yaw_ref   - Yaw reference command (-1 to 1)
%   alt_ref   - Altitude/Throttle reference command (0 to 1)
%
% Outputs:
%   M1_PWM to M4_PWM - Motor PWM signals (0 to 1)
%
% Motor configuration (X-frame):
%   M1(Front Right)    M4(Front Left)
%          \           /
%           \         /
%            \ === /
%            / === \
%           /         \
%          /           \
%   M2(Back Right)    M3(Back Left)

% Mixing matrix for X configuration
% For positive roll: M3,M4 increase, M1,M2 decrease
% For positive pitch: M1,M4 increase, M2,M3 decrease
% For positive yaw: M1,M3 increase, M2,M4 decrease
% For altitude: all motors increase equally

% Motor mixing computation
M4_PWM = alt_ref + roll_ref + pitch_ref - yaw_ref;   % Front Left
M3_PWM = alt_ref + roll_ref - pitch_ref + yaw_ref;   % Back Left
M2_PWM = alt_ref - roll_ref - pitch_ref - yaw_ref;   % Back Right
M1_PWM = alt_ref - roll_ref + pitch_ref + yaw_ref;   % Front Right

% Constrain outputs between 0 and 1
M4_PWM = min(max(M4_PWM, 0), 1);
M3_PWM = min(max(M3_PWM, 0), 1);
M2_PWM = min(max(M2_PWM, 0), 1);
M1_PWM = min(max(M1_PWM, 0), 1);

== matlab function drone_1/BLDC_Motor2/BLDC_Dynamics ==
  settings: updateMethod=DISCRETE
  data: Veff input; omega output; torque output; thrust output
function [omega, torque, thrust] = fcn(Veff)
%#codegen
% Simplified BLDC Motor and Propeller Dynamics for Quadcopter
% Input:
%   Veff - Effective voltage from ESC (V)
% Outputs:
%   omega - Motor angular velocity (rad/s)
%   torque - Motor torque (N*m)
%   thrust - Propeller thrust (N)

% Motor Parameters (based on your drone mass and inertia data)
Kv = 920;                  % Motor velocity constant (RPM/V)
Km = 60/(Kv*2*pi);        % Motor torque constant (N*m/A)
R = 0.1;                  % Motor resistance (ohm)
J = 1.915e-3;            % Rotor inertia from provided data (kg*m^2)
B = 1e-5;                % Viscous damping coefficient (N*m*s)

% Propeller Parameters
Ct = 1.2e-6;             % Thrust coefficient
Cq = 1.8e-7;             % Torque coefficient
rho = 1.225;             % Air density (kg/m^3)
D = 0.254;               % Propeller diameter (m)

% Motor Speed Calculation
% Using steady-state approximation
omega = (Veff - 0)/(Km^2/R + B);  % Steady state speed

% Torque Calculation
current = (Veff - Km*omega)/R;
aero_torque = Cq*rho*D^5*omega^2;
torque = Km*current - B*omega - aero_torque;

% Thrust Calculation
thrust = Ct*rho*D^4*omega^2;

% Limit minimum speed/thrust for numerical stability
if omega < 0
    omega = 0;
    torque = 0;
    thrust = 0;
end
end

== matlab function drone_1/BLDC_Motor2/ESC_Logic ==
  data: pwm_input input; Veff output
function Veff = fcn(pwm_input)
%#codegen
% Simplified ESC Logic for BLDC Motor Control
% Input:
%   pwm_input - PWM signal (0 to 1)
% Output:
%   Veff - Effective voltage to motor (V)

% ESC Parameters
MIN_THROTTLE = 0.05;        % Minimum throttle (deadband)
MAX_THROTTLE = 0.95;        % Maximum throttle limit
BATTERY_VOLTAGE = 14.8;     % Assuming 4S LiPo (14.8V)

% Apply deadband
if pwm_input < MIN_THROTTLE
    normalized_pwm = 0;
elseif pwm_input > MAX_THROTTLE
    normalized_pwm = 1;
else
    % Normalize PWM to 0-1 range considering deadband
    normalized_pwm = (pwm_input - MIN_THROTTLE) / (MAX_THROTTLE - MIN_THROTTLE);
end

% Convert to effective voltage
Veff = BATTERY_VOLTAGE * normalized_pwm;
end

== matlab function drone_1/BLDC_Motor3/BLDC_Dynamics ==
  settings: updateMethod=DISCRETE
  data: Veff input; omega output; torque output; thrust output
function [omega, torque, thrust] = fcn(Veff)
%#codegen
% Simplified BLDC Motor and Propeller Dynamics for Quadcopter
% Input:
%   Veff - Effective voltage from ESC (V)
% Outputs:
%   omega - Motor angular velocity (rad/s)
%   torque - Motor torque (N*m)
%   thrust - Propeller thrust (N)

% Motor Parameters (based on your drone mass and inertia data)
Kv = 920;                  % Motor velocity constant (RPM/V)
Km = 60/(Kv*2*pi);        % Motor torque constant (N*m/A)
R = 0.1;                  % Motor resistance (ohm)
J = 1.915e-3;            % Rotor inertia from provided data (kg*m^2)
B = 1e-5;                % Viscous damping coefficient (N*m*s)

% Propeller Parameters
Ct = 1.2e-6;             % Thrust coefficient
Cq = 1.8e-7;             % Torque coefficient
rho = 1.225;             % Air density (kg/m^3)
D = 0.254;               % Propeller diameter (m)

% Motor Speed Calculation
% Using steady-state approximation
omega = (Veff - 0)/(Km^2/R + B);  % Steady state speed

% Torque Calculation
current = (Veff - Km*omega)/R;
aero_torque = Cq*rho*D^5*omega^2;
torque = Km*current - B*omega - aero_torque;

% Thrust Calculation
thrust = Ct*rho*D^4*omega^2;

% Limit minimum speed/thrust for numerical stability
if omega < 0
    omega = 0;
    torque = 0;
    thrust = 0;
end
end

== matlab function drone_1/BLDC_Motor3/ESC_Logic ==
  data: pwm_input input; Veff output
function Veff = fcn(pwm_input)
%#codegen
% Simplified ESC Logic for BLDC Motor Control
% Input:
%   pwm_input - PWM signal (0 to 1)
% Output:
%   Veff - Effective voltage to motor (V)

% ESC Parameters
MIN_THROTTLE = 0.05;        % Minimum throttle (deadband)
MAX_THROTTLE = 0.95;        % Maximum throttle limit
BATTERY_VOLTAGE = 14.8;     % Assuming 4S LiPo (14.8V)

% Apply deadband
if pwm_input < MIN_THROTTLE
    normalized_pwm = 0;
elseif pwm_input > MAX_THROTTLE
    normalized_pwm = 1;
else
    % Normalize PWM to 0-1 range considering deadband
    normalized_pwm = (pwm_input - MIN_THROTTLE) / (MAX_THROTTLE - MIN_THROTTLE);
end

% Convert to effective voltage
Veff = BATTERY_VOLTAGE * normalized_pwm;
end

== matlab function drone_1/BLDC_Motor4/BLDC_Dynamics ==
  settings: updateMethod=DISCRETE
  data: Veff input; omega output; torque output; thrust output
function [omega, torque, thrust] = fcn(Veff)
%#codegen
% Simplified BLDC Motor and Propeller Dynamics for Quadcopter
% Input:
%   Veff - Effective voltage from ESC (V)
% Outputs:
%   omega - Motor angular velocity (rad/s)
%   torque - Motor torque (N*m)
%   thrust - Propeller thrust (N)

% Motor Parameters (based on your drone mass and inertia data)
Kv = 920;                  % Motor velocity constant (RPM/V)
Km = 60/(Kv*2*pi);        % Motor torque constant (N*m/A)
R = 0.1;                  % Motor resistance (ohm)
J = 1.915e-3;            % Rotor inertia from provided data (kg*m^2)
B = 1e-5;                % Viscous damping coefficient (N*m*s)

% Propeller Parameters
Ct = 1.2e-6;             % Thrust coefficient
Cq = 1.8e-7;             % Torque coefficient
rho = 1.225;             % Air density (kg/m^3)
D = 0.254;               % Propeller diameter (m)

% Motor Speed Calculation
% Using steady-state approximation
omega = (Veff - 0)/(Km^2/R + B);  % Steady state speed

% Torque Calculation
current = (Veff - Km*omega)/R;
aero_torque = Cq*rho*D^5*omega^2;
torque = Km*current - B*omega - aero_torque;

% Thrust Calculation
thrust = Ct*rho*D^4*omega^2;

% Limit minimum speed/thrust for numerical stability
if omega < 0
    omega = 0;
    torque = 0;
    thrust = 0;
end
end

== matlab function drone_1/BLDC_Motor4/ESC_Logic ==
  data: pwm_input input; Veff output
function Veff = fcn(pwm_input)
%#codegen
% Simplified ESC Logic for BLDC Motor Control
% Input:
%   pwm_input - PWM signal (0 to 1)
% Output:
%   Veff - Effective voltage to motor (V)

% ESC Parameters
MIN_THROTTLE = 0.05;        % Minimum throttle (deadband)
MAX_THROTTLE = 0.95;        % Maximum throttle limit
BATTERY_VOLTAGE = 14.8;     % Assuming 4S LiPo (14.8V)

% Apply deadband
if pwm_input < MIN_THROTTLE
    normalized_pwm = 0;
elseif pwm_input > MAX_THROTTLE
    normalized_pwm = 1;
else
    % Normalize PWM to 0-1 range considering deadband
    normalized_pwm = (pwm_input - MIN_THROTTLE) / (MAX_THROTTLE - MIN_THROTTLE);
end

% Convert to effective voltage
Veff = BATTERY_VOLTAGE * normalized_pwm;
end
